simulink model "SPGF_FSK_0000_R2022b"  (R2022b)
settings: Solver=ode4  StartTime=0.0  StopTime=1.4  FixedStep=50e-6/50  RelTol=1e-3  EnableMultiTasking=on
undefined symbols (not defined in the file): D11, Delta
libraries: spsSeriesRLCBranchLib x1646, spsGroundLib x360, spsStairGeneratorLib x147, spsIdealSwitchLib x145, spsCurrentMeasurementLib x145, spsUniversalBridgeLib x76, spsThreePhaseSeriesRLCLoadLib x57, simulink x45, spsBistableLib x36, spsSequenceAnalyzerLib x31, spsThreePhaseParallelRLCLoadLib x20, spsThreePhaseTransformerTwoWindingsLib x20
(part 21 of 40)

== system SPGF_FSK_0000_R2022b/W15/concentrated ==
  Ccs/1 : spsSeriesRLCBranchLib/Series RLC Branch  LConnTagsString=__new0  RConnTagsString=__new0  BranchType=C  Resistance=190  Inductance=1e-3  SetiL0=off  InitialCurrent=0  Capacitance=-C_matrix(1,2)/2  Setx0=off  InitialVoltage=0  Measurements=None
  Ccs/2 : spsSeriesRLCBranchLib/Series RLC Branch  LConnTagsString=__new0  RConnTagsString=__new0  BranchType=C  Resistance=190  Inductance=1e-3  SetiL0=off  InitialCurrent=0  Capacitance=-C_matrix(1,2)/2  Setx0=off  InitialVoltage=0  Measurements=None
  Ccs2/1 : spsSeriesRLCBranchLib/Series RLC Branch  LConnTagsString=__new0  RConnTagsString=__new0  BranchType=C  Resistance=190  Inductance=1e-3  SetiL0=off  InitialCurrent=0  Capacitance=-C_matrix(3,4)/2  Setx0=off  InitialVoltage=0  Measurements=None
  Ccs2/2 : spsSeriesRLCBranchLib/Series RLC Branch  LConnTagsString=__new0  RConnTagsString=__new0  BranchType=C  Resistance=190  Inductance=1e-3  SetiL0=off  InitialCurrent=0  Capacitance=-C_matrix(3,4)/2  Setx0=off  InitialVoltage=0  Measurements=None
  Ccs2/3 : spsSeriesRLCBranchLib/Series RLC Branch  LConnTagsString=__new0  RConnTagsString=__new0  BranchType=R  Resistance=-Rg_matrix(3,4)*2  Inductance=1e-3  SetiL0=off  InitialCurrent=0  Capacitance=Rg_matrix(3,4)*2  Setx0=off  InitialVoltage=0  Measurements=None
  Ccs2/4 : spsSeriesRLCBranchLib/Series RLC Branch  LConnTagsString=__new0  RConnTagsString=__new0  BranchType=R  Resistance=-Rg_matrix(3,4)*2  Inductance=1e-3  SetiL0=off  InitialCurrent=0  Capacitance=Rg_matrix(3,4)*2  Setx0=off  InitialVoltage=0  Measurements=None
  Ccs3/1 : spsSeriesRLCBranchLib/Series RLC Branch  LConnTagsString=__new0  RConnTagsString=__new0  BranchType=C  Resistance=190  Inductance=1e-3  SetiL0=off  InitialCurrent=0  Capacitance=-C_matrix(5,6)/2  Setx0=off  InitialVoltage=0  Measurements=None
  Ccs3/2 : spsSeriesRLCBranchLib/Series RLC Branch  LConnTagsString=__new0  RConnTagsString=__new0  BranchType=C  Resistance=190  Inductance=1e-3  SetiL0=off  InitialCurrent=0  Capacitance=-C_matrix(5,6)/2  Setx0=off  InitialVoltage=0  Measurements=None
  Ccs3/3 : spsSeriesRLCBranchLib/Series RLC Branch  LConnTagsString=__new0  RConnTagsString=__new0  BranchType=R  Resistance=-Rg_matrix(5,6)*2  Inductance=1e-3  SetiL0=off  InitialCurrent=0  Capacitance=-C_matrix(5,6)/2  Setx0=off  InitialVoltage=0  Measurements=None
  Ccs3/4 : spsSeriesRLCBranchLib/Series RLC Branch  LConnTagsString=__new0  RConnTagsString=__new0  BranchType=R  Resistance=-Rg_matrix(5,6)*2  Inductance=1e-3  SetiL0=off  InitialCurrent=0  Capacitance=-C_matrix(5,6)/2  Setx0=off  InitialVoltage=0  Measurements=None
  Csg/2 : spsSeriesRLCBranchLib/Series RLC Branch  LConnTagsString=__new0  RConnTagsString=__new0  BranchType=C  Resistance=190  Inductance=1e-3  SetiL0=off  InitialCurrent=0  Capacitance=( C_matrix(1,2) + C_matrix(2,2) )/2  Setx0=off  InitialVoltage=0  Measurements=None
  Csg1/1 : spsSeriesRLCBranchLib/Series RLC Branch  LConnTagsString=__new0  RConnTagsString=__new0  BranchType=C  Resistance=190  Inductance=1e-3  SetiL0=off  InitialCurrent=0  Capacitance=( C_matrix(1,2) + C_matrix(2,2) )/2  Setx0=off  InitialVoltage=0  Measurements=None
  Csg2/1 : spsSeriesRLCBranchLib/Series RLC Branch  LConnTagsString=__new0  RConnTagsString=__new0  BranchType=C  Resistance=190  Inductance=1e-3  SetiL0=off  InitialCurrent=0  Capacitance=( C_matrix(3,4) + C_matrix(4,4) )/2  Setx0=off  InitialVoltage=0  Measurements=None
  Csg2/2 : spsSeriesRLCBranchLib/Series RLC Branch  LConnTagsString=__new0  RConnTagsString=__new0  BranchType=C  Resistance=190  Inductance=1e-3  SetiL0=off  InitialCurrent=0  Capacitance=( C_matrix(3,4) + C_matrix(4,4) )/2  Setx0=off  InitialVoltage=0  Measurements=None
  Csg3/1 : spsSeriesRLCBranchLib/Series RLC Branch  LConnTagsString=__new0  RConnTagsString=__new0  BranchType=C  Resistance=190  Inductance=1e-3  SetiL0=off  InitialCurrent=0  Capacitance=( C_matrix(5,6) + C_matrix(6,6) ) /2  Setx0=off  InitialVoltage=0  Measurements=None
  Csg3/2 : spsSeriesRLCBranchLib/Series RLC Branch  LConnTagsString=__new0  RConnTagsString=__new0  BranchType=C  Resistance=190  Inductance=1e-3  SetiL0=off  InitialCurrent=0  Capacitance=( C_matrix(5,6) + C_matrix(6,6) ) /2  Setx0=off  InitialVoltage=0  Measurements=None
  Ground{1..4} (4 alike) : spsGroundLib/Ground  LConnTagsString=a
  RL : spsMutualInductanceLib/Mutual Inductance  LConnTagsString=a|b|c|L4|L5|L6  RConnTagsString=A|B|C|R4|R5|R6  TypeOfMutual=Generalized mutual inductance  NumberOfWindings=6  SelfImpedance1=[1.1 1.1e-03]  SelfImpedance2=[ 1.1 1.1e-03]  ThreeWindings=on  SelfImpedance3=[ 1.1 1.1e-03]  MutualImpedance=[1.0 1.0e-03]  InductanceMatrix=L_matrix  ResistanceMatrix=R_matrix  Measurements=None
      settings: LibrarySourceBlock=sps_lib/Passives/Mutual Inductance
  Rcs*2 : spsSeriesRLCBranchLib/Series RLC Branch  LConnTagsString=__new0  RConnTagsString=__new0  BranchType=R  Resistance=-Rg_matrix(1,2)*2  Inductance=1e-3  SetiL0=off  InitialCurrent=0  Capacitance=Rg_matrix(1,2)*2  Setx0=off  InitialVoltage=0  Measurements=None
  Rgcs1/1 : spsSeriesRLCBranchLib/Series RLC Branch  LConnTagsString=__new0  RConnTagsString=__new0  BranchType=R  Resistance=-Rg_matrix(1,2)*2  Inductance=1e-3  SetiL0=off  InitialCurrent=0  Capacitance=Rg_matrix(1,2)*2  Setx0=off  InitialVoltage=0  Measurements=None
  Rgsg1/1 : spsSeriesRLCBranchLib/Series RLC Branch  LConnTagsString=__new0  RConnTagsString=__new0  BranchType=R  Resistance=(Rg_matrix(4,4)+Rg_matrix(3,4))*2  Inductance=1e-3  SetiL0=off  InitialCurrent=0  Capacitance=Rg_matrix(1,2)*2  Setx0=off  InitialVoltage=0  Measurements=None
  Rgsg1/2 : spsSeriesRLCBranchLib/Series RLC Branch  LConnTagsString=__new0  RConnTagsString=__new0  BranchType=R  Resistance=(Rg_matrix(2,2)+Rg_matrix(1,2))*2  Inductance=1e-3  SetiL0=off  InitialCurrent=0  Capacitance=Rg_matrix(1,2)*2  Setx0=off  InitialVoltage=0  Measurements=None
  Rgsg1/3 : spsSeriesRLCBranchLib/Series RLC Branch  LConnTagsString=__new0  RConnTagsString=__new0  BranchType=R  Resistance=(Rg_matrix(4,4)+Rg_matrix(3,4))*2  Inductance=1e-3  SetiL0=off  InitialCurrent=0  Capacitance=Rg_matrix(1,2)*2  Setx0=off  InitialVoltage=0  Measurements=None
  Rgsg1/4 : spsSeriesRLCBranchLib/Series RLC Branch  LConnTagsString=__new0  RConnTagsString=__new0  BranchType=R  Resistance=(Rg_matrix(2,2)+Rg_matrix(1,2))*2  Inductance=1e-3  SetiL0=off  InitialCurrent=0  Capacitance=Rg_matrix(1,2)*2  Setx0=off  InitialVoltage=0  Measurements=None
  Rsg*2 : spsSeriesRLCBranchLib/Series RLC Branch  LConnTagsString=__new0  RConnTagsString=__new0  BranchType=R  Resistance=(Rg_matrix(6,6)+Rg_matrix(5,6))*2  Inductance=1e-3  SetiL0=off  InitialCurrent=0  Capacitance=Rg_matrix(1,2)*2  Setx0=off  InitialVoltage=0  Measurements=None
  Rsg1/1 : spsSeriesRLCBranchLib/Series RLC Branch  LConnTagsString=__new0  RConnTagsString=__new0  BranchType=R  Resistance=(Rg_matrix(6,6)+Rg_matrix(5,6))*2  Inductance=1e-3  SetiL0=off  InitialCurrent=0  Capacitance=Rg_matrix(1,2)*2  Setx0=off  InitialVoltage=0  Measurements=None
  A : PMIOPort  Side=Left
  B : PMIOPort  Port=2  Side=Left
  C : PMIOPort  Port=3  Side=Left
  a : PMIOPort  Port=4  Side=Right
  b : PMIOPort  Port=5  Side=Right
  c : PMIOPort  Port=6  Side=Right
  connections:
  Ccs3/3/RConn1 -- RL/LConn5 -- C/RConn1 -- Ccs3/2/RConn1
  Ccs2/2/RConn1 -- Ccs2/3/RConn1 -- B/RConn1 -- RL/LConn3
  Ccs/2/RConn1 -- Rcs*2/RConn1 -- A/RConn1 -- RL/LConn1
  Ccs3/4/RConn1 -- RL/RConn5 -- c/RConn1 -- Ccs3/1/RConn1
  Ccs2/1/RConn1 -- Ccs2/4/RConn1 -- RL/RConn3 -- b/RConn1
  Ccs/1/RConn1 -- Rgcs1/1/RConn1 -- RL/RConn1 -- a/RConn1
  Csg/2/RConn1 -- Ground1/LConn1 -- Csg2/2/RConn1 -- Csg3/2/RConn1 -- Rgsg1/2/RConn1 -- Rgsg1/1/RConn1 -- Rsg*2/RConn1
  Csg3/1/LConn1 -- Ccs3/4/LConn1 -- Rsg1/1/LConn1 -- Ccs3/1/LConn1 -- RL/RConn6 -- Ground4/LConn1 -- RL/RConn2 -- Ccs/1/LConn1 -- Csg1/1/LConn1 -- Rgcs1/1/LConn1 -- Rgsg1/4/LConn1 -- RL/RConn4 -- Ccs2/1/LConn1 -- Csg2/1/LConn1 -- Ccs2/4/LConn1 -- Rgsg1/3/LConn1
  Csg1/1/RConn1 -- Ground2/LConn1 -- Csg2/1/RConn1 -- Csg3/1/RConn1 -- Rgsg1/4/RConn1 -- Rgsg1/3/RConn1 -- Rsg1/1/RConn1
  Ccs3/2/LConn1 -- Ccs3/3/LConn1 -- Csg3/2/LConn1 -- Rsg*2/LConn1 -- Ccs2/2/LConn1 -- Ccs2/3/LConn1 -- Csg2/2/LConn1 -- Rgsg1/1/LConn1 -- RL/LConn4 -- RL/LConn2 -- Ccs/2/LConn1 -- Rcs*2/LConn1 -- Csg/2/LConn1 -- Rgsg1/2/LConn1 -- Ground3/LConn1 -- RL/LConn6

== system SPGF_FSK_0000_R2022b/W21/DPL ==
  Ccs2/1 : spsSeriesRLCBranchLib/Series RLC Branch  LConnTagsString=__new0  RConnTagsString=__new0  BranchType=R  Resistance=-Rg_matrix(3,4)*2  Inductance=1e-3  SetiL0=off  InitialCurrent=0  Capacitance=Rg_matrix(3,4)*2  Setx0=off  InitialVoltage=0  Measurements=None
  Ccs2/3 : spsSeriesRLCBranchLib/Series RLC Branch  LConnTagsString=__new0  RConnTagsString=__new0  BranchType=R  Resistance=-Rg_matrix(3,4)*2  Inductance=1e-3  SetiL0=off  InitialCurrent=0  Capacitance=Rg_matrix(3,4)*2  Setx0=off  InitialVoltage=0  Measurements=None
  Ccs3/1 : spsSeriesRLCBranchLib/Series RLC Branch  LConnTagsString=__new0  RConnTagsString=__new0  BranchType=R  Resistance=-Rg_matrix(5,6)*2  Inductance=1e-3  SetiL0=off  InitialCurrent=0  Capacitance=-C_matrix(5,6)/2  Setx0=off  InitialVoltage=0  Measurements=None
  Ccs3/3 : spsSeriesRLCBranchLib/Series RLC Branch  LConnTagsString=__new0  RConnTagsString=__new0  BranchType=R  Resistance=-Rg_matrix(5,6)*2  Inductance=1e-3  SetiL0=off  InitialCurrent=0  Capacitance=-C_matrix(5,6)/2  Setx0=off  InitialVoltage=0  Measurements=None
  DPL : spsDistributedParametersLineLib/Distributed Parameters Line  Phases=6  Length=LineLength  Frequency=Frequency  Resistance=R_matrix  Inductance=L_matrix  Capacitance=C_matrix  x1=[-2.8e-05 -1.16534888629937 5056.85583270413 0 -2770.28944118531 0 0;-2.75e-05 -1.16569158516128 5058.29147397259 0 -2771.07592630165 0 0;-2.7e-05 -1.1660342552609 5059.72699043271 0 -2771.86234304442 0 0;-2.65e-05 -1.16637689658978 5061.16238204907 0 -2772.64869139424 0 0;-2.6e-05 -1.16671950913946 5062.59764878626 0 -2773.43497133169 0 0;-2.55e-05 -1.16706209290149 5064.03279060886 0 -2774.22118283738 0 0;-2.5e-05 -1.16740464786742 5065.46780748145 0 -2775.00732589191 0 0;-2.45e-05 -1.16774717402879 5066.90269936864 0 -2775.79340047587 0 0;-2.4e-05 -1.16808967137715 5068.33746623502 0 -2776.57940656987 0 0;-2.35e-05 -1.16843213990406 5069.77210804518 0 -2777.36534415453 0 0;-2.3e-05 -1.16877457960107 5071.20662476372 0 -2778.15121321044 0 0;-2.25e-05 -1.16911699045971 5072.64101635526 0 -2778.93701371822 0 0;-2.2e-05 -1.16945937247155 5074.07528278441 0 -2779.72274565848 0 0;-2.15e-05 -1.16980172562814 5075.50942401576 0 -2780.50840901182 0 0;-2.1e-05 -1.17014404992102 5076.94344001393 0 -2781.29400375888 0 0;-2.05e-05 -1.17048634534176 5078.37733074355 0 -2782.07952988025 0 0;-2e-05 -1.1708286118819 5079.81109616923 0 -2782.86498735656 0 0;-1.95e-05 -1.17117084953301 5081.2447362556 0 -2783.65037616843 0 0;-1.9e-05 -1.17151305828664 5082.67825096728 0 -2784.43569629649 0 0;-1.85e-05 -1.17185523813434 5084.1116402689 0 -2785.22094772134 0 0;-1.8e-05 -1.17219738906767 5085.54490412509 0 -2786.00613042362 0 0;-1.75e-05 -1.17253951107819 5086.97804250049 0 -2786.79124438396 0 0;-1.7e-05 -1.17288160415745 5088.41105535974 0 -2787.57628958298 0 0;-1.65e-05 -1.17322366829702 5089.84394266748 0 -2788.36126600131 0 0;-1.6e-05 -1.17356570348846 5091.27670438835 0 -2789.14617361959 0 0;-1.55e-05 -1.17390770972333 5092.70934048701 0 -2789.93101241844 0 0;-1.5e-05 -1.17424968699318 5094.1418509281 0 -2790.7157823785 0 0;-1.45e-05 -1.17459163528959 5095.57423567628 0 -2791.50048348041 0 0;-1.4e-05 -1.1749335546041 5097.00649469621 0 -2792.28511570481 0 0;-1.35e-05 -1.1752754449283 5098.43862795254 0 -2793.06967903233 0 0;-1.3e-05 -1.17561730625373 5099.87063540994 0 -2793.85417344363 0 0;-1.25e-05 -1.17595913857198 5101.30251703308 0 -2794.63859891933 0 0;-1.2e-05 -1.17630094187459 5102.73427278662 0 -2795.42295544009 0 0;-1.15e-05 -1.17664271615314 5104.16590263524 0 -2796.20724298656 0 0;-1.1e-05 -1.17698446139919 5105.59740654362 0 -2796.99146153937 0 0;-1.05e-05 -1.17732617760432 5107.02878447643 0 -2797.77561107919 0 0;-1e-05 -1.17766786476009 5108.46003639835 0 -2798.55969158666 0 0;-9.5e-06 -1.17800952285806 5109.89116227408 0 -2799.34370304244 0 0;-9e-06 -1.17835115188982 5111.32216206829 0 -2800.12764542718 0 0;-8.5e-06 -1.17869275184693 5112.75303574569 0 -2800.91151872155 0 0;-8e-06 -1.17903432272096 5114.18378327096 0 -2801.69532290619 0 0;-7.5e-06 -1.17937586450349 5115.61440460881 0 -2802.47905796177 0 0;-7e-06 -1.17971737718608 5117.04489972393 0 -2803.26272386895 0 0;-6.5e-06 -1.18005886076032 5118.47526858103 0 -2804.04632060839 0 0;-6e-06 -1.18040031521776 5119.90551114481 0 -2804.82984816077 0 0;-5.5e-06 -1.18074174055 5121.33562737999 -12.6660829679671 -2805.61330650674 0 0;-5e-06 -1.1810831367486 5122.76561725128 -12.6698010202153 -2806.39669562698 0 0;-4.5e-06 -1.18142450380515 5124.19548072339 -12.6735187598487 -2807.18001550216 4987.30313046272 -9097.9489590017;-4e-06 -1.18176584171121 5125.62521776104 -12.6772361867756 -2807.96326611294 4986.86192214537 -9097.14409700584;-3.5e-06 -1.18210715045837 5127.05482832897 -12.6809533009042 -2808.74644744002 4986.42059078213 -9096.33901054695;-3e-06 -1.18244843003821 5128.48431239189 -12.6846701021429 -2809.52955946405 4985.9791363839 -9095.53369964489;-2.5e-06 -1.1827896804423 5129.91366991452 -12.6883865903998 -2810.31260216571 4985.53755896156 -9094.72816431953;-2e-06 -1.18313090166222 5131.34290086162 -12.6921027655834 -2811.09557552569 4985.09585852602 -9093.92240459075;-1.5e-06 -1.18347209368956 5132.7720051979 -12.6958186276018 -2811.87847952467 4984.65403508816 -9093.11642047843;-1e-06 -1.1838132565159 5134.20098288811 -12.6995341763636 -2812.66131414333 4984.2120886589 -9092.31021200245;-5e-07 -1.18415439013281 5135.62983389699 -12.7032494117768 -2813.44407936236 4983.77001924914 -9091.50377918271]  x2=[-2.8e-05 -1.16510912460452 5063.16244321356 0 -2773.74438176613 0 0;-2.75e-05 -1.16545352542046 5064.60090637248 0 -2774.53241279433 0 0;-2.7e-05 -1.16579789747999 5066.03924456738 0 -2775.32037536367 0 0;-2.65e-05 -1.1661422407746 5067.47745776277 0 -2776.10826945474 0 0;-2.6e-05 -1.16648655529581 5068.91554592317 0 -2776.89609504807 0 0;-2.55e-05 -1.16683084103512 5070.35350901309 0 -2777.68385212425 0 0;-2.5e-05 -1.16717509798403 5071.79134699705 0 -2778.47154066382 0 0;-2.45e-05 -1.16751932613405 5073.22905983957 0 -2779.25916064735 0 0;-2.4e-05 -1.16786352547669 5074.66664750519 0 -2780.04671205541 0 0;-2.35e-05 -1.16820769600344 5076.10410995842 0 -2780.83419486857 0 0;-2.3e-05 -1.16855183770583 5077.54144716381 0 -2781.6216090674 0 0;-2.25e-05 -1.16889595057536 5078.97865908588 0 -2782.40895463246 0 0;-2.2e-05 -1.16924003460353 5080.41574568918 0 -2783.19623154434 0 0;-2.15e-05 -1.16958408978187 5081.85270693825 0 -2783.9834397836 0 0;-2.1e-05 -1.16992811610187 5083.28954279763 0 -2784.77057933082 0 0;-2.05e-05 -1.17027211355506 5084.72625323186 0 -2785.55765016658 0 0;-2e-05 -1.17061608213293 5086.1628382055 0 -2786.34465227147 0 0;-1.95e-05 -1.17096002182702 5087.59929768311 0 -2787.13158562605 0 0;-1.9e-05 -1.17130393262882 5089.03563162923 0 -2787.91845021092 0 0;-1.85e-05 -1.17164781452986 5090.47184000843 0 -2788.70524600666 0 0;-1.8e-05 -1.17199166752164 5091.90792278528 0 -2789.49197299386 0 0;-1.75e-05 -1.17233549159569 5093.34387992433 0 -2790.2786311531 0 0;-1.7e-05 -1.17267928674353 5094.77971139016 0 -2791.06522046497 0 0;-1.65e-05 -1.17302305295666 5096.21541714735 0 -2791.85174091007 0 0;-1.6e-05 -1.1733667902266 5097.65099716045 0 -2792.63819246899 0 0;-1.55e-05 -1.17371049854489 5099.08645139406 0 -2793.42457512233 0 0;-1.5e-05 -1.17405417790302 5100.52177981275 0 -2794.21088885067 0 0;-1.45e-05 -1.17439782829253 5101.95698238112 0 -2794.99713363463 0 0;-1.4e-05 -1.17474144970494 5103.39205906374 0 -2795.78330945479 0 0;-1.35e-05 -1.17508504213176 5104.82700982521 0 -2796.56941629177 0 0;-1.3e-05 -1.17542860556452 5106.26183463012 0 -2797.35545412617 0 0;-1.25e-05 -1.17577213999474 5107.69653344307 0 -2798.14142293858 0 0;-1.2e-05 -1.17611564541395 5109.13110622866 0 -2798.92732270962 0 0;-1.15e-05 -1.17645912181367 5110.5655529515 0 -2799.7131534199 0 0;-1.1e-05 -1.17680256918542 5111.99987357618 0 -2800.49891505003 0 0;-1.05e-05 -1.17714598752073 5113.43406806733 0 -2801.28460758061 0 0;-1e-05 -1.17748937681113 5114.86813638954 0 -2802.07023099227 0 0;-9.5e-06 -1.17783273704815 5116.30207850745 0 -2802.85578526562 0 0;-9e-06 -1.1781760682233 5117.73589438565 0 -2803.64127038127 0 0;-8.5e-06 -1.17851937032813 5119.16958398879 0 -2804.42668631985 0 0;-8e-06 -1.17886264335416 5120.60314728148 0 -2805.21203306197 0 0;-7.5e-06 -1.17920588729292 5122.03658422836 0 -2805.99731058826 0 0;-7e-06 -1.17954910213593 5123.46989479404 0 -2806.78251887934 0 0;-6.5e-06 -1.17989228787475 5124.90307894318 0 -2807.56765791584 0 0;-6e-06 -1.18023544450088 5126.3361366404 0 -2808.35272767838 0 0;-5.5e-06 -1.18057857200588 5127.76906785034 -12.6564826349605 -2809.1377281476 0 0;-5e-06 -1.18092167038126 5129.20187253766 -12.6602239684602 -2809.92265930412 0 0;-4.5e-06 -1.18126473961857 5130.63455066699 -12.6639649895814 -2810.70752112858 4996.71752818238 -9115.12291207668;-4e-06 -1.18160777970934 5132.06710220299 -12.6677056982318 -2811.49231360161 4996.27596698537 -9114.31740634991;-3.5e-06 -1.18195079064511 5133.49952711031 -12.6714460943191 -2812.27703670385 4995.83428251018 -9113.51167573637;-3e-06 -1.18229377241741 5134.9318253536 -12.675186177751 -2813.06169041594 4995.39247476773 -9112.70572025595;-2.5e-06 -1.18263672501778 5136.36399689754 -12.6789259484352 -2813.84627471851 4994.95054376891 -9111.89953992853;-2e-06 -1.18297964843776 5137.79604170677 -12.6826654062795 -2814.6307895922 4994.50848952462 -9111.09313477399;-1.5e-06 -1.18332254266889 5139.22795974596 -12.6864045511915 -2815.41523501767 4994.06631204578 -9110.28650481225;-1e-06 -1.18366540770271 5140.65975097979 -12.6901433830791 -2816.19961097555 4993.62401134329 -9109.4796500632;-5e-07 -1.18400824353075 5142.09141537292 -12.6938819018499 -2816.98391744649 4993.18158742807 -9108.67257054674]  x3=[-2.8e-05 -4.26783627359743e-06 43.4620546748687 0 -260.320398510763 0 0;-2.75e-05 -6.64716416284354e-06 43.4958297492458 0 -260.396991199751 0 0;-2.7e-05 -9.0264918880775e-06 43.5296037504063 0 -260.473577463702 0 0;-2.65e-05 -1.14058193905917e-05 43.5633766775169 0 -260.550157300724 0 0;-2.6e-05 -1.37851466116785e-05 43.5971485297442 0 -260.626730708929 0 0;-2.55e-05 -1.61644734926305e-05 43.630919306255 0 -260.703297686428 0 0;-2.5e-05 -1.85437999747402e-05 43.664689006216 0 -260.77985823133 0 0;-2.45e-05 -2.09231259992999e-05 43.6984576287941 0 -260.856412341747 0 0;-2.4e-05 -2.33024515076021e-05 43.7322251731559 0 -260.93296001579 0 0;-2.35e-05 -2.56817764409394e-05 43.7659916384683 0 -261.00950125157 0 0;-2.3e-05 -2.80611007406043e-05 43.7997570238981 0 -261.0860360472 0 0;-2.25e-05 -3.04404243478893e-05 43.8335213286123 0 -261.162564400789 0 0;-2.2e-05 -3.28197472040869e-05 43.8672845517776 0 -261.23908631045 0 0;-2.15e-05 -3.51990692504896e-05 43.9010466925612 0 -261.315601774296 0 0;-2.1e-05 -3.75783904283902e-05 43.9348077501298 0 -261.392110790437 0 0;-2.05e-05 -3.99577106790812e-05 43.9685677236505 0 -261.468613356987 0 0;-2e-05 -4.23370299438552e-05 44.0023266122902 0 -261.545109472057 0 0;-1.95e-05 -4.47163481640048e-05 44.0360844152161 0 -261.62159913376 0 0;-1.9e-05 -4.70956652808228e-05 44.0698411315951 0 -261.698082340209 0 0;-1.85e-05 -4.94749812356017e-05 44.1035967605944 0 -261.774559089517 0 0;-1.8e-05 -5.18542959696346e-05 44.1373513013811 0 -261.851029379796 0 0;-1.75e-05 -5.42336094242139e-05 44.1711047531223 0 -261.92749320916 0 0;-1.7e-05 -5.66129215406325e-05 44.2048571149851 0 -262.003950575723 0 0;-1.65e-05 -5.89922322601833e-05 44.2386083861368 0 -262.080401477597 0 0;-1.6e-05 -6.13715415241591e-05 44.2723585657447 0 -262.156845912896 0 0;-1.55e-05 -6.37508492738528e-05 44.3061076529758 0 -262.233283879734 0 0;-1.5e-05 -6.61301554505574e-05 44.3398556469976 0 -262.309715376226 0 0;-1.45e-05 -6.85094599955658e-05 44.3736025469773 0 -262.386140400484 0 0;-1.4e-05 -7.0888762850171e-05 44.4073483520822 0 -262.462558950625 0 0;-1.35e-05 -7.32680639556661e-05 44.4410930614798 0 -262.538971024761 0 0;-1.3e-05 -7.56473632533442e-05 44.4748366743373 0 -262.615376621007 0 0;-1.25e-05 -7.80266606844984e-05 44.5085791898222 0 -262.691775737479 0 0;-1.2e-05 -8.0405956190422e-05 44.5423206071019 0 -262.768168372292 0 0;-1.15e-05 -8.27852497124081e-05 44.576060925344 0 -262.844554523559 0 0;-1.1e-05 -8.516454119175e-05 44.6098001437158 0 -262.920934189397 0 0;-1.05e-05 -8.75438305697411e-05 44.6435382613849 0 -262.997307367922 0 0;-1e-05 -8.99231177876749e-05 44.6772752775189 0 -263.073674057247 0 0;-9.5e-06 -9.23024027868445e-05 44.7110111912853 0 -263.15003425549 0 0;-9e-06 -9.46816855085437e-05 44.7447460018517 0 -263.226387960766 0 0;-8.5e-06 -9.7060965894066e-05 44.7784797083857 0 -263.302735171192 0 0;-8e-06 -9.94402438847049e-05 44.8122123100551 0 -263.379075884883 0 0;-7.5e-06 -0.000101819519421754 44.8459438060274 0 -263.455410099955 0 0;-7e-06 -0.000104198792446507 44.8796741954705 0 -263.531737814526 0 0;-6.5e-06 -0.000106578062900259 44.9134034775519 0 -263.608059026712 0 0;-6e-06 -0.000108957330724302 44.9471316514396 0 -263.68437373463 0 0;-5.5e-06 -0.00011133659585993 44.9808587163012 -0.835958382231405 -263.760681936397 0 0;-5e-06 -0.000113715858248438 45.0145846713046 -0.836322757975905 -263.83698363013 0 0;-4.5e-06 -0.00011609511783112 45.0483095156177 -0.836687113084968 -263.913278813946 514.841663054707 -236.599753323224;-4e-06 -0.00011847437454927 45.0820332484083 -0.837051447549604 -263.989567485963 514.798101260749 -236.590465344622;-3.5e-06 -0.000120853628344181 45.1157558688443 -0.837415761360824 -264.065849644298 514.754526764657 -236.581171528384;-3e-06 -0.000123232879157149 45.1494773760937 -0.837780054509638 -264.14212528707 514.710939567506 -236.571871874739;-2.5e-06 -0.000125612126929467 45.1831977693243 -0.838144326987057 -264.218394412396 514.667339670372 -236.562566383918 ...(+471 chars)]  x4=[-2.8e-05 -0.0140226628107478 91.5383252097823 0 -240.863301074738 0 0;-2.75e-05 -0.0140244628801063 91.5429574729256 0 -240.929298928784 0 0;-2.7e-05 -0.0140262626034252 91.5475874773368 0 -240.995290838137 0 0;-2.65e-05 -0.0140280619806598 91.552215222902 0 -241.061276801169 0 0;-2.6e-05 -0.0140298610117659 91.5568407095068 0 -241.127256816253 0 0;-2.55e-05 -0.0140316596966991 91.561463937037 0 -241.193230881761 0 0;-2.5e-05 -0.014033458035415 91.5660849053787 0 -241.259198996064 0 0;-2.45e-05 -0.0140352560278691 91.5707036144179 0 -241.325161157535 0 0;-2.4e-05 -0.0140370536740172 91.5753200640405 0 -241.391117364546 0 0;-2.35e-05 -0.0140388509738149 91.5799342541326 0 -241.45706761547 0 0;-2.3e-05 -0.0140406479272178 91.5845461845804 0 -241.52301190868 0 0;-2.25e-05 -0.0140424445341816 91.5891558552702 0 -241.588950242549 0 0;-2.2e-05 -0.014044240794662 91.5937632660881 0 -241.654882615449 0 0;-2.15e-05 -0.0140460367086146 91.5983684169205 0 -241.720809025754 0 0;-2.1e-05 -0.0140478322759951 91.6029713076537 0 -241.786729471837 0 0;-2.05e-05 -0.0140496274967593 91.6075719381743 0 -241.852643952071 0 0;-2e-05 -0.0140514223708629 91.6121703083685 0 -241.918552464831 0 0;-1.95e-05 -0.0140532168982615 91.6167664181231 0 -241.984455008489 0 0;-1.9e-05 -0.0140550110789108 91.6213602673247 0 -242.050351581421 0 0;-1.85e-05 -0.0140568049127667 91.6259518558597 0 -242.116242182 0 0;-1.8e-05 -0.0140585983997848 91.630541183615 0 -242.182126808599 0 0;-1.75e-05 -0.0140603915399209 91.6351282504774 0 -242.248005459595 0 0;-1.7e-05 -0.0140621843331307 91.6397130563335 0 -242.31387813336 0 0;-1.65e-05 -0.01406397677937 91.6442956010704 0 -242.37974482827 0 0;-1.6e-05 -0.0140657688785947 91.648875884575 0 -242.4456055427 0 0;-1.55e-05 -0.0140675606307603 91.6534539067342 0 -242.511460275024 0 0;-1.5e-05 -0.0140693520358229 91.658029667435 0 -242.577309023618 0 0;-1.45e-05 -0.0140711430937381 91.6626031665647 0 -242.643151786856 0 0;-1.4e-05 -0.0140729338044618 91.6671744040102 0 -242.708988563115 0 0;-1.35e-05 -0.0140747241679497 91.6717433796589 0 -242.774819350769 0 0;-1.3e-05 -0.0140765141841577 91.676310093398 0 -242.840644148195 0 0;-1.25e-05 -0.0140783038530417 91.6808745451148 0 -242.906462953769 0 0;-1.2e-05 -0.0140800931745575 91.6854367346967 0 -242.972275765865 0 0;-1.15e-05 -0.0140818821486608 91.6899966620311 0 -243.038082582861 0 0;-1.1e-05 -0.0140836707753077 91.6945543270055 0 -243.103883403133 0 0;-1.05e-05 -0.0140854590544539 91.6991097295076 0 -243.169678225056 0 0;-1e-05 -0.0140872469860554 91.7036628694247 0 -243.235467047009 0 0;-9.5e-06 -0.0140890345700679 91.7082137466447 0 -243.301249867366 0 0;-9e-06 -0.0140908218064475 91.7127623610553 0 -243.367026684507 0 0;-8.5e-06 -0.01409260869515 91.7173087125441 0 -243.432797496806 0 0;-8e-06 -0.0140943952361313 91.721852800999 0 -243.498562302642 0 0;-7.5e-06 -0.0140961814293473 91.726394626308 0 -243.564321100392 0 0;-7e-06 -0.014097967274754 91.7309341883588 0 -243.630073888433 0 0;-6.5e-06 -0.0140997527723073 91.7354714870396 0 -243.695820665142 0 0;-6e-06 -0.0141015379219631 91.7400065222384 0 -243.761561428899 0 0;-5.5e-06 -0.0141033227236775 91.7445392938432 -1.0186771696074 -243.82729617808 0 0;-5e-06 -0.0141051071774063 91.7490698017423 -1.01886024502449 -243.893024911064 0 0;-4.5e-06 -0.0141068912831055 91.7535980458238 -1.01904329530221 -243.958747626228 450.89936877339 -48.814783490625;-4e-06 -0.0141086750407311 91.7581240259761 -1.01922632043605 -244.024464321952 450.857682085038 -48.7988728473647;-3.5e-06 -0.0141104584502392 91.7626477420874 -1.01940932042148 -244.090174996614 450.815984272219 -48.7829610000405;-3e-06 -0.0141122415115856 91.7671691940461 -1.019592295254 -244.155879648591 450.774275335962 -48.767047949045;-2.5e-06 -0.0141140242247264 91.7716883817406 -1.01977524492909 -244.221578276264 450.732555277295 -48.7511336947708;-2e-06 -0.0141158065896177 91.7762053050596 -1.01995816944223 -244.287270878011 450.690824097248 -48.7352182376106;-1.5e-06 -0.0141175886062154 91.7807199638914 -1.02014106878891 -244.352957452212 450.649081796851 -48.7193015779571;-1e-06 -0.0141193702744755 91.7852323581247 -1.02032394296462 -244.418637997244 450.607328377133 -48.7033837162031;-5e-07 -0.0141211515943542 91.7897424876483 -1.02050679196485 -244.484312511489 450.565563839125 -48.6874646527412]  x5=2.77139177619252e-05  V1=ones(3,3)  V2=ones(3,3)  I1=ones(3,3)  I2=ones(3,3)  nHarmo=1  Measurements=None  Decoupling=off  VsMag0=0  VrMag0=0  VsAngle0=0  VrAngle0=0  IsMag0=0  IrMag0=0  IsAngle0=0  IrAngle0=0
      settings: LibrarySourceBlock=sps_lib/Power Grid Elements/Distributed Parameters Line
  Ground{1..4} (4 alike) : spsGroundLib/Ground  LConnTagsString=a
  Rcs*1 : spsSeriesRLCBranchLib/Series RLC Branch  LConnTagsString=__new0  RConnTagsString=__new0  BranchType=R  Resistance=-Rg_matrix(1,2)*2  Inductance=1e-3  SetiL0=off  InitialCurrent=0  Capacitance=Rg_matrix(1,2)*2  Setx0=off  InitialVoltage=0  Measurements=None
  Rcs*2 : spsSeriesRLCBranchLib/Series RLC Branch  LConnTagsString=__new0  RConnTagsString=__new0  BranchType=R  Resistance=-Rg_matrix(1,2)*2  Inductance=1e-3  SetiL0=off  InitialCurrent=0  Capacitance=Rg_matrix(1,2)*2  Setx0=off  InitialVoltage=0  Measurements=None
  Rgsg1/1 : spsSeriesRLCBranchLib/Series RLC Branch  LConnTagsString=__new0  RConnTagsString=__new0  BranchType=R  Resistance=(Rg_matrix(4,4)+Rg_matrix(3,4))*2  Inductance=1e-3  SetiL0=off  InitialCurrent=0  Capacitance=Rg_matrix(1,2)*2  Setx0=off  InitialVoltage=0  Measurements=None
  Rgsg1/2 : spsSeriesRLCBranchLib/Series RLC Branch  LConnTagsString=__new0  RConnTagsString=__new0  BranchType=R  Resistance=(Rg_matrix(2,2)+Rg_matrix(1,2))*2  Inductance=1e-3  SetiL0=off  InitialCurrent=0  Capacitance=Rg_matrix(1,2)*2  Setx0=off  InitialVoltage=0  Measurements=None
  Rgsg1/3 : spsSeriesRLCBranchLib/Series RLC Branch  LConnTagsString=__new0  RConnTagsString=__new0  BranchType=R  Resistance=(Rg_matrix(4,4)+Rg_matrix(3,4))*2  Inductance=1e-3  SetiL0=off  InitialCurrent=0  Capacitance=Rg_matrix(1,2)*2  Setx0=off  InitialVoltage=0  Measurements=None
  Rgsg1/4 : spsSeriesRLCBranchLib/Series RLC Branch  LConnTagsString=__new0  RConnTagsString=__new0  BranchType=R  Resistance=(Rg_matrix(2,2)+Rg_matrix(1,2))*2  Inductance=1e-3  SetiL0=off  InitialCurrent=0  Capacitance=Rg_matrix(1,2)*2  Setx0=off  InitialVoltage=0  Measurements=None
  Rsg*1 : spsSeriesRLCBranchLib/Series RLC Branch  LConnTagsString=__new0  RConnTagsString=__new0  BranchType=R  Resistance=(Rg_matrix(6,6)+Rg_matrix(5,6))*2  Inductance=1e-3  SetiL0=off  InitialCurrent=0  Capacitance=Rg_matrix(1,2)*2  Setx0=off  InitialVoltage=0  Measurements=None
  Rsg*2 : spsSeriesRLCBranchLib/Series RLC Branch  LConnTagsString=__new0  RConnTagsString=__new0  BranchType=R  Resistance=(Rg_matrix(6,6)+Rg_matrix(5,6))*2  Inductance=1e-3  SetiL0=off  InitialCurrent=0  Capacitance=Rg_matrix(1,2)*2  Setx0=off  InitialVoltage=0  Measurements=None
  A : PMIOPort  Side=Left
  B : PMIOPort  Port=2  Side=Left
  C : PMIOPort  Port=3  Side=Left
  a : PMIOPort  Port=4  Side=Right
  b : PMIOPort  Port=5  Side=Right
  c : PMIOPort  Port=6  Side=Right
  connections:
  A/RConn1 -- DPL/LConn1 -- Rcs*2/RConn1
  B/RConn1 -- DPL/LConn3 -- Ccs2/3/RConn1
  C/RConn1 -- DPL/LConn5 -- Ccs3/3/RConn1
  Rgsg1/2/RConn1 -- Rsg*2/RConn1 -- Rgsg1/1/RConn1 -- Ground2/LConn1
  DPL/LConn2 -- Rcs*2/LConn1 -- Rgsg1/2/LConn1 -- DPL/LConn4 -- Ccs2/3/LConn1 -- Rgsg1/1/LConn1 -- DPL/LConn6 -- Rsg*2/LConn1 -- Ccs3/3/LConn1 -- Ground3/LConn1
  Rgsg1/3/RConn1 -- Rsg*1/RConn1 -- Rgsg1/4/RConn1 -- Ground1/LConn1
  Rgsg1/3/LConn1 -- Ccs2/1/LConn1 -- DPL/RConn4 -- DPL/RConn2 -- Rgsg1/4/LConn1 -- Rcs*1/LConn1 -- Rsg*1/LConn1 -- Ccs3/1/LConn1 -- DPL/RConn6 -- Ground4/LConn1
  Rcs*1/RConn1 -- DPL/RConn1 -- a/RConn1
  DPL/RConn3 -- Ccs2/1/RConn1 -- b/RConn1
  DPL/RConn5 -- Ccs3/1/RConn1 -- c/RConn1

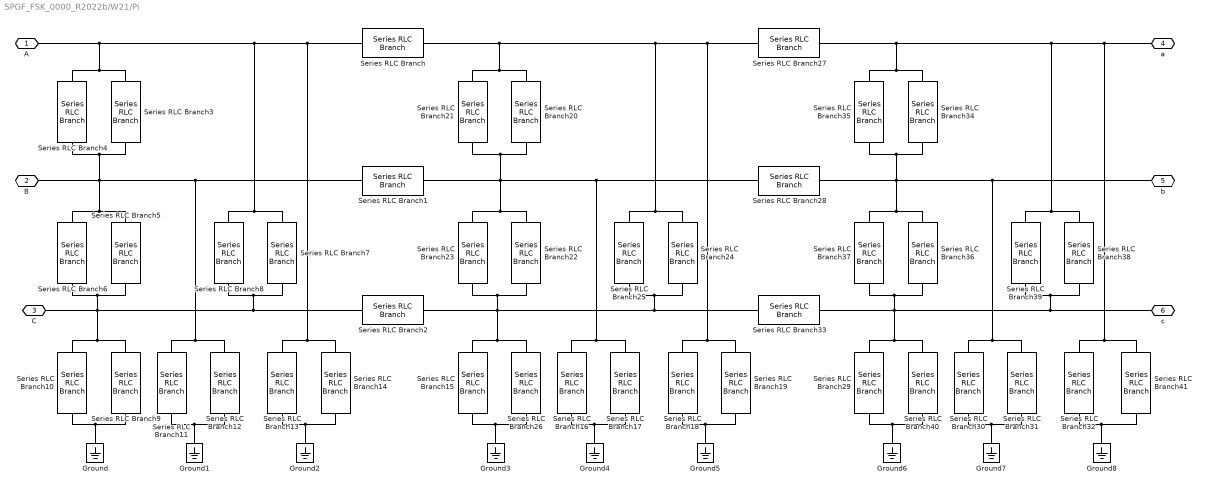
== system SPGF_FSK_0000_R2022b/W21/Pi ==
  Ground{,1..8} (9 alike) : spsGroundLib/Ground  LConnTagsString=a
  Series RLC Branch{,1..2,27..28,33} (6 alike) : spsSeriesRLCBranchLib/Series RLC Branch  LConnTagsString=__new0  RConnTagsString=__new0  BranchType=RL  Resistance=R/2  Inductance=L/2  SetiL0=off  InitialCurrent=0  Capacitance=1e-6  Setx0=off  InitialVoltage=0  Measurements=None
  Series RLC Branch{10..11,13,29..30,32} (6 alike) : spsSeriesRLCBranchLib/Series RLC Branch  LConnTagsString=__new0  RConnTagsString=__new0  BranchType=R  Resistance=Rfg*4  Inductance=L/2  SetiL0=off  InitialCurrent=0  Capacitance=1e-6  Setx0=off  InitialVoltage=0  Measurements=None
  Series RLC Branch{9,12,14,31,40..41} (6 alike) : spsSeriesRLCBranchLib/Series RLC Branch  LConnTagsString=__new0  RConnTagsString=__new0  BranchType=C  Resistance=R/2  Inductance=L/2  SetiL0=off  InitialCurrent=0  Capacitance=Cfg*0.25  Setx0=off  InitialVoltage=0  Measurements=None
  Series RLC Branch15 : spsSeriesRLCBranchLib/Series RLC Branch  LConnTagsString=__new0  RConnTagsString=__new0  BranchType=R  Resistance=Rfg*2  Inductance=L/2  SetiL0=off  InitialCurrent=0  Capacitance=1e-6  Setx0=off  InitialVoltage=0  Measurements=None
  Series RLC Branch16 : spsSeriesRLCBranchLib/Series RLC Branch  LConnTagsString=__new0  RConnTagsString=__new0  BranchType=R  Resistance=Rfg*2  Inductance=L/2  SetiL0=off  InitialCurrent=0  Capacitance=1e-6  Setx0=off  InitialVoltage=0  Measurements=None
  Series RLC Branch17 : spsSeriesRLCBranchLib/Series RLC Branch  LConnTagsString=__new0  RConnTagsString=__new0  BranchType=C  Resistance=R/2  Inductance=L/2  SetiL0=off  InitialCurrent=0  Capacitance=Cfg*0.5  Setx0=off  InitialVoltage=0  Measurements=None
  Series RLC Branch18 : spsSeriesRLCBranchLib/Series RLC Branch  LConnTagsString=__new0  RConnTagsString=__new0  BranchType=R  Resistance=Rfg*2  Inductance=L/2  SetiL0=off  InitialCurrent=0  Capacitance=1e-6  Setx0=off  InitialVoltage=0  Measurements=None
  Series RLC Branch19 : spsSeriesRLCBranchLib/Series RLC Branch  LConnTagsString=__new0  RConnTagsString=__new0  BranchType=C  Resistance=R/2  Inductance=L/2  SetiL0=off  InitialCurrent=0  Capacitance=Cfg*0.5  Setx0=off  InitialVoltage=0  Measurements=None
  Series RLC Branch20 : spsSeriesRLCBranchLib/Series RLC Branch  LConnTagsString=__new0  RConnTagsString=__new0  BranchType=C  Resistance=R/2  Inductance=L/2  SetiL0=off  InitialCurrent=0  Capacitance=Cmf*0.5  Setx0=off  InitialVoltage=0  Measurements=None
  Series RLC Branch21 : spsSeriesRLCBranchLib/Series RLC Branch  LConnTagsString=__new0  RConnTagsString=__new0  BranchType=R  Resistance=Rmf*2  Inductance=L/2  SetiL0=off  InitialCurrent=0  Capacitance=1e-6  Setx0=off  InitialVoltage=0  Measurements=None
  Series RLC Branch22 : spsSeriesRLCBranchLib/Series RLC Branch  LConnTagsString=__new0  RConnTagsString=__new0  BranchType=C  Resistance=R/2  Inductance=L/2  SetiL0=off  InitialCurrent=0  Capacitance=Cmf*0.5  Setx0=off  InitialVoltage=0  Measurements=None
  Series RLC Branch23 : spsSeriesRLCBranchLib/Series RLC Branch  LConnTagsString=__new0  RConnTagsString=__new0  BranchType=R  Resistance=Rmf*2  Inductance=L/2  SetiL0=off  InitialCurrent=0  Capacitance=1e-6  Setx0=off  InitialVoltage=0  Measurements=None
  Series RLC Branch24 : spsSeriesRLCBranchLib/Series RLC Branch  LConnTagsString=__new0  RConnTagsString=__new0  BranchType=C  Resistance=R/2  Inductance=L/2  SetiL0=off  InitialCurrent=0  Capacitance=Cmf*0.5  Setx0=off  InitialVoltage=0  Measurements=None
  Series RLC Branch25 : spsSeriesRLCBranchLib/Series RLC Branch  LConnTagsString=__new0  RConnTagsString=__new0  BranchType=R  Resistance=Rmf*2  Inductance=L/2  SetiL0=off  InitialCurrent=0  Capacitance=1e-6  Setx0=off  InitialVoltage=0  Measurements=None
  Series RLC Branch26 : spsSeriesRLCBranchLib/Series RLC Branch  LConnTagsString=__new0  RConnTagsString=__new0  BranchType=C  Resistance=R/2  Inductance=L/2  SetiL0=off  InitialCurrent=0  Capacitance=Cfg*0.5  Setx0=off  InitialVoltage=0  Measurements=None
  Series RLC Branch{3,5,7,34,36,38} (6 alike) : spsSeriesRLCBranchLib/Series RLC Branch  LConnTagsString=__new0  RConnTagsString=__new0  BranchType=C  Resistance=R/2  Inductance=L/2  SetiL0=off  InitialCurrent=0  Capacitance=Cmf*0.25  Setx0=off  InitialVoltage=0  Measurements=None
  Series RLC Branch{4,6,8,35,37,39} (6 alike) : spsSeriesRLCBranchLib/Series RLC Branch  LConnTagsString=__new0  RConnTagsString=__new0  BranchType=R  Resistance=Rmf*4  Inductance=L/2  SetiL0=off  InitialCurrent=0  Capacitance=1e-6  Setx0=off  InitialVoltage=0  Measurements=None
  A : PMIOPort  Side=Left
  B : PMIOPort  Port=2  Side=Left
  C : PMIOPort  Port=3  Side=Left
  a : PMIOPort  Port=4  Side=Right
  b : PMIOPort  Port=5  Side=Right
  c : PMIOPort  Port=6  Side=Right
  connections:
  Series RLC Branch12/LConn1 -- Series RLC Branch11/LConn1 -- Series RLC Branch5/LConn1 -- Series RLC Branch6/LConn1 -- B/RConn1 -- Series RLC Branch4/RConn1 -- Series RLC Branch3/RConn1 -- Series RLC Branch1/LConn1
  Series RLC Branch13/LConn1 -- A/RConn1 -- Series RLC Branch4/LConn1 -- Series RLC Branch3/LConn1 -- Series RLC Branch7/LConn1 -- Series RLC Branch8/LConn1 -- Series RLC Branch/LConn1 -- Series RLC Branch14/LConn1
  Series RLC Branch9/LConn1 -- Series RLC Branch2/LConn1 -- Series RLC Branch8/RConn1 -- Series RLC Branch7/RConn1 -- C/RConn1 -- Series RLC Branch5/RConn1 -- Series RLC Branch6/RConn1 -- Series RLC Branch10/LConn1
  Series RLC Branch9/RConn1 -- Ground/LConn1 -- Series RLC Branch10/RConn1
  Series RLC Branch12/RConn1 -- Series RLC Branch11/RConn1 -- Ground1/LConn1
  Series RLC Branch13/RConn1 -- Series RLC Branch14/RConn1 -- Ground2/LConn1
  Series RLC Branch17/LConn1 -- Series RLC Branch16/LConn1 -- Series RLC Branch28/LConn1 -- Series RLC Branch1/RConn1 -- Series RLC Branch23/LConn1 -- Series RLC Branch22/LConn1 -- Series RLC Branch20/RConn1 -- Series RLC Branch21/RConn1
  Series RLC Branch21/LConn1 -- Series RLC Branch20/LConn1 -- Series RLC Branch/RConn1 -- Series RLC Branch27/LConn1 -- Series RLC Branch19/LConn1 -- Series RLC Branch18/LConn1 -- Series RLC Branch24/LConn1 -- Series RLC Branch25/LConn1
  Series RLC Branch26/LConn1 -- Series RLC Branch15/LConn1 -- Series RLC Branch2/RConn1 -- Series RLC Branch33/LConn1 -- Series RLC Branch25/RConn1 -- Series RLC Branch24/RConn1 -- Series RLC Branch22/RConn1 -- Series RLC Branch23/RConn1
  Series RLC Branch26/RConn1 -- Series RLC Branch15/RConn1 -- Ground3/LConn1
  Ground4/LConn1 -- Series RLC Branch17/RConn1 -- Series RLC Branch16/RConn1
  Ground5/LConn1 -- Series RLC Branch18/RConn1 -- Series RLC Branch19/RConn1
  Series RLC Branch31/LConn1 -- b/RConn1 -- Series RLC Branch35/RConn1 -- Series RLC Branch34/RConn1 -- Series RLC Branch36/LConn1 -- Series RLC Branch37/LConn1 -- Series RLC Branch28/RConn1 -- Series RLC Branch30/LConn1
  Series RLC Branch34/LConn1 -- a/RConn1 -- Series RLC Branch41/LConn1 -- Series RLC Branch32/LConn1 -- Series RLC Branch38/LConn1 -- Series RLC Branch39/LConn1 -- Series RLC Branch27/RConn1 -- Series RLC Branch35/LConn1
  Series RLC Branch29/LConn1 -- Series RLC Branch36/RConn1 -- Series RLC Branch37/RConn1 -- c/RConn1 -- Series RLC Branch39/RConn1 -- Series RLC Branch38/RConn1 -- Series RLC Branch33/RConn1 -- Series RLC Branch40/LConn1
  Series RLC Branch29/RConn1 -- Series RLC Branch40/RConn1 -- Ground6/LConn1
  Series RLC Branch31/RConn1 -- Series RLC Branch30/RConn1 -- Ground7/LConn1
  Series RLC Branch32/RConn1 -- Series RLC Branch41/RConn1 -- Ground8/LConn1

== system SPGF_FSK_0000_R2022b/W21/Q ==
  breaker : Subsystem  Commented=on  mask{SwitchA=on, SwitchB=on, SwitchC=on, InitialStatus=[0 0 0], BreakerResistance=0.0001, SnubberResistance=1e6, SnubberCapacitance=inf, TransitionTimes=[0.2], ShiftTimes=[0 0.02 0.04]}
      mask prompts: SwitchA "Switching of phase A"; SwitchB "Switching of phase B"; SwitchC "Switching of phase C"; InitialStatus "Initial status of phase breaker [A, B, C]"; BreakerResistance "Breaker resistance Ron (ohms) :"; SnubberResistance "Snubbers resistance Rp (ohms) :"; SnubberCapacitance "Snubbers capacitance Cp (F) :"; TransitionTimes "Transition times (s) :"; ShiftTimes "Time differences for switch [tA, tB, tC] (s) :"
      mask init: same as SPGF_FSK_0000_R2022b/Feed/Q/breaker
      mask Display:
      | % port_label('input',1,'Iabc');
      | 
      | port_label('lconn',1,'A');
      | port_label('lconn',2,'B');
      | port_label('lconn',3,'C');
      | 
      | port_label('rconn',1,'a');
      | port_label('rconn',2,'b');
      | port_label('rconn',3,'c');
      | 
      | disp('   Q    ');
  meas : Subsystem
  shunt : Subsystem
  A : PMIOPort  Side=Right
  B : PMIOPort  Port=2  Side=Right
  C : PMIOPort  Port=3  Side=Right
  a : PMIOPort  Port=4  Side=Left
  b : PMIOPort  Port=5  Side=Left
  c : PMIOPort  Port=6  Side=Left
  connections:
  shunt/LConn3 -- breaker/LConn3 -- C/RConn1
  shunt/LConn2 -- breaker/LConn2 -- B/RConn1
  A/RConn1 -- breaker/LConn1 -- shunt/LConn1
  meas/RConn1 -- a/RConn1
  meas/RConn2 -- b/RConn1
  meas/RConn3 -- c/RConn1
  meas/LConn3 -- breaker/RConn3 -- shunt/RConn3
  meas/LConn2 -- breaker/RConn2 -- shunt/RConn2
  meas/LConn1 -- breaker/RConn1 -- shunt/RConn1

== system SPGF_FSK_0000_R2022b/W21/concentrated ==
  Ccs/1 : spsSeriesRLCBranchLib/Series RLC Branch  LConnTagsString=__new0  RConnTagsString=__new0  BranchType=C  Resistance=190  Inductance=1e-3  SetiL0=off  InitialCurrent=0  Capacitance=-C_matrix(1,2)/2  Setx0=off  InitialVoltage=0  Measurements=None
  Ccs/2 : spsSeriesRLCBranchLib/Series RLC Branch  LConnTagsString=__new0  RConnTagsString=__new0  BranchType=C  Resistance=190  Inductance=1e-3  SetiL0=off  InitialCurrent=0  Capacitance=-C_matrix(1,2)/2  Setx0=off  InitialVoltage=0  Measurements=None
  Ccs2/1 : spsSeriesRLCBranchLib/Series RLC Branch  LConnTagsString=__new0  RConnTagsString=__new0  BranchType=C  Resistance=190  Inductance=1e-3  SetiL0=off  InitialCurrent=0  Capacitance=-C_matrix(3,4)/2  Setx0=off  InitialVoltage=0  Measurements=None
  Ccs2/2 : spsSeriesRLCBranchLib/Series RLC Branch  LConnTagsString=__new0  RConnTagsString=__new0  BranchType=C  Resistance=190  Inductance=1e-3  SetiL0=off  InitialCurrent=0  Capacitance=-C_matrix(3,4)/2  Setx0=off  InitialVoltage=0  Measurements=None
  Ccs2/3 : spsSeriesRLCBranchLib/Series RLC Branch  LConnTagsString=__new0  RConnTagsString=__new0  BranchType=R  Resistance=-Rg_matrix(3,4)*2  Inductance=1e-3  SetiL0=off  InitialCurrent=0  Capacitance=Rg_matrix(3,4)*2  Setx0=off  InitialVoltage=0  Measurements=None
  Ccs2/4 : spsSeriesRLCBranchLib/Series RLC Branch  LConnTagsString=__new0  RConnTagsString=__new0  BranchType=R  Resistance=-Rg_matrix(3,4)*2  Inductance=1e-3  SetiL0=off  InitialCurrent=0  Capacitance=Rg_matrix(3,4)*2  Setx0=off  InitialVoltage=0  Measurements=None
  Ccs3/1 : spsSeriesRLCBranchLib/Series RLC Branch  LConnTagsString=__new0  RConnTagsString=__new0  BranchType=C  Resistance=190  Inductance=1e-3  SetiL0=off  InitialCurrent=0  Capacitance=-C_matrix(5,6)/2  Setx0=off  InitialVoltage=0  Measurements=None
  Ccs3/2 : spsSeriesRLCBranchLib/Series RLC Branch  LConnTagsString=__new0  RConnTagsString=__new0  BranchType=C  Resistance=190  Inductance=1e-3  SetiL0=off  InitialCurrent=0  Capacitance=-C_matrix(5,6)/2  Setx0=off  InitialVoltage=0  Measurements=None
  Ccs3/3 : spsSeriesRLCBranchLib/Series RLC Branch  LConnTagsString=__new0  RConnTagsString=__new0  BranchType=R  Resistance=-Rg_matrix(5,6)*2  Inductance=1e-3  SetiL0=off  InitialCurrent=0  Capacitance=-C_matrix(5,6)/2  Setx0=off  InitialVoltage=0  Measurements=None
  Ccs3/4 : spsSeriesRLCBranchLib/Series RLC Branch  LConnTagsString=__new0  RConnTagsString=__new0  BranchType=R  Resistance=-Rg_matrix(5,6)*2  Inductance=1e-3  SetiL0=off  InitialCurrent=0  Capacitance=-C_matrix(5,6)/2  Setx0=off  InitialVoltage=0  Measurements=None
  Csg/2 : spsSeriesRLCBranchLib/Series RLC Branch  LConnTagsString=__new0  RConnTagsString=__new0  BranchType=C  Resistance=190  Inductance=1e-3  SetiL0=off  InitialCurrent=0  Capacitance=( C_matrix(1,2) + C_matrix(2,2) )/2  Setx0=off  InitialVoltage=0  Measurements=None
  Csg1/1 : spsSeriesRLCBranchLib/Series RLC Branch  LConnTagsString=__new0  RConnTagsString=__new0  BranchType=C  Resistance=190  Inductance=1e-3  SetiL0=off  InitialCurrent=0  Capacitance=( C_matrix(1,2) + C_matrix(2,2) )/2  Setx0=off  InitialVoltage=0  Measurements=None
  Csg2/1 : spsSeriesRLCBranchLib/Series RLC Branch  LConnTagsString=__new0  RConnTagsString=__new0  BranchType=C  Resistance=190  Inductance=1e-3  SetiL0=off  InitialCurrent=0  Capacitance=( C_matrix(3,4) + C_matrix(4,4) )/2  Setx0=off  InitialVoltage=0  Measurements=None
  Csg2/2 : spsSeriesRLCBranchLib/Series RLC Branch  LConnTagsString=__new0  RConnTagsString=__new0  BranchType=C  Resistance=190  Inductance=1e-3  SetiL0=off  InitialCurrent=0  Capacitance=( C_matrix(3,4) + C_matrix(4,4) )/2  Setx0=off  InitialVoltage=0  Measurements=None
  Csg3/1 : spsSeriesRLCBranchLib/Series RLC Branch  LConnTagsString=__new0  RConnTagsString=__new0  BranchType=C  Resistance=190  Inductance=1e-3  SetiL0=off  InitialCurrent=0  Capacitance=( C_matrix(5,6) + C_matrix(6,6) ) /2  Setx0=off  InitialVoltage=0  Measurements=None
  Csg3/2 : spsSeriesRLCBranchLib/Series RLC Branch  LConnTagsString=__new0  RConnTagsString=__new0  BranchType=C  Resistance=190  Inductance=1e-3  SetiL0=off  InitialCurrent=0  Capacitance=( C_matrix(5,6) + C_matrix(6,6) ) /2  Setx0=off  InitialVoltage=0  Measurements=None
  Ground{1..4} (4 alike) : spsGroundLib/Ground  LConnTagsString=a
  RL : spsMutualInductanceLib/Mutual Inductance  LConnTagsString=a|b|c|L4|L5|L6  RConnTagsString=A|B|C|R4|R5|R6  TypeOfMutual=Generalized mutual inductance  NumberOfWindings=6  SelfImpedance1=[1.1 1.1e-03]  SelfImpedance2=[ 1.1 1.1e-03]  ThreeWindings=on  SelfImpedance3=[ 1.1 1.1e-03]  MutualImpedance=[1.0 1.0e-03]  InductanceMatrix=L_matrix  ResistanceMatrix=R_matrix  Measurements=None
      settings: LibrarySourceBlock=sps_lib/Passives/Mutual Inductance
  Rcs*2 : spsSeriesRLCBranchLib/Series RLC Branch  LConnTagsString=__new0  RConnTagsString=__new0  BranchType=R  Resistance=-Rg_matrix(1,2)*2  Inductance=1e-3  SetiL0=off  InitialCurrent=0  Capacitance=Rg_matrix(1,2)*2  Setx0=off  InitialVoltage=0  Measurements=None
  Rgcs1/1 : spsSeriesRLCBranchLib/Series RLC Branch  LConnTagsString=__new0  RConnTagsString=__new0  BranchType=R  Resistance=-Rg_matrix(1,2)*2  Inductance=1e-3  SetiL0=off  InitialCurrent=0  Capacitance=Rg_matrix(1,2)*2  Setx0=off  InitialVoltage=0  Measurements=None
  Rgsg1/1 : spsSeriesRLCBranchLib/Series RLC Branch  LConnTagsString=__new0  RConnTagsString=__new0  BranchType=R  Resistance=(Rg_matrix(4,4)+Rg_matrix(3,4))*2  Inductance=1e-3  SetiL0=off  InitialCurrent=0  Capacitance=Rg_matrix(1,2)*2  Setx0=off  InitialVoltage=0  Measurements=None
  Rgsg1/2 : spsSeriesRLCBranchLib/Series RLC Branch  LConnTagsString=__new0  RConnTagsString=__new0  BranchType=R  Resistance=(Rg_matrix(2,2)+Rg_matrix(1,2))*2  Inductance=1e-3  SetiL0=off  InitialCurrent=0  Capacitance=Rg_matrix(1,2)*2  Setx0=off  InitialVoltage=0  Measurements=None
  Rgsg1/3 : spsSeriesRLCBranchLib/Series RLC Branch  LConnTagsString=__new0  RConnTagsString=__new0  BranchType=R  Resistance=(Rg_matrix(4,4)+Rg_matrix(3,4))*2  Inductance=1e-3  SetiL0=off  InitialCurrent=0  Capacitance=Rg_matrix(1,2)*2  Setx0=off  InitialVoltage=0  Measurements=None
  Rgsg1/4 : spsSeriesRLCBranchLib/Series RLC Branch  LConnTagsString=__new0  RConnTagsString=__new0  BranchType=R  Resistance=(Rg_matrix(2,2)+Rg_matrix(1,2))*2  Inductance=1e-3  SetiL0=off  InitialCurrent=0  Capacitance=Rg_matrix(1,2)*2  Setx0=off  InitialVoltage=0  Measurements=None
  Rsg*2 : spsSeriesRLCBranchLib/Series RLC Branch  LConnTagsString=__new0  RConnTagsString=__new0  BranchType=R  Resistance=(Rg_matrix(6,6)+Rg_matrix(5,6))*2  Inductance=1e-3  SetiL0=off  InitialCurrent=0  Capacitance=Rg_matrix(1,2)*2  Setx0=off  InitialVoltage=0  Measurements=None
  Rsg1/1 : spsSeriesRLCBranchLib/Series RLC Branch  LConnTagsString=__new0  RConnTagsString=__new0  BranchType=R  Resistance=(Rg_matrix(6,6)+Rg_matrix(5,6))*2  Inductance=1e-3  SetiL0=off  InitialCurrent=0  Capacitance=Rg_matrix(1,2)*2  Setx0=off  InitialVoltage=0  Measurements=None
  A : PMIOPort  Side=Left
  B : PMIOPort  Port=2  Side=Left
  C : PMIOPort  Port=3  Side=Left
  a : PMIOPort  Port=4  Side=Right
  b : PMIOPort  Port=5  Side=Right
  c : PMIOPort  Port=6  Side=Right
  connections:
  RL/LConn6 -- Ground3/LConn1 -- Rgsg1/2/LConn1 -- Csg/2/LConn1 -- Rcs*2/LConn1 -- Ccs/2/LConn1 -- RL/LConn2 -- RL/LConn4 -- Rgsg1/1/LConn1 -- Csg2/2/LConn1 -- Ccs2/3/LConn1 -- Ccs2/2/LConn1 -- Rsg*2/LConn1 -- Csg3/2/LConn1 -- Ccs3/3/LConn1 -- Ccs3/2/LConn1
  Rsg1/1/RConn1 -- Rgsg1/3/RConn1 -- Rgsg1/4/RConn1 -- Csg3/1/RConn1 -- Csg2/1/RConn1 -- Ground2/LConn1 -- Csg1/1/RConn1
  Rgsg1/3/LConn1 -- Ccs2/4/LConn1 -- Csg2/1/LConn1 -- Ccs2/1/LConn1 -- RL/RConn4 -- Rgsg1/4/LConn1 -- Rgcs1/1/LConn1 -- Csg1/1/LConn1 -- Ccs/1/LConn1 -- RL/RConn2 -- Ground4/LConn1 -- RL/RConn6 -- Ccs3/1/LConn1 -- Rsg1/1/LConn1 -- Ccs3/4/LConn1 -- Csg3/1/LConn1
  Rsg*2/RConn1 -- Rgsg1/1/RConn1 -- Rgsg1/2/RConn1 -- Csg3/2/RConn1 -- Csg2/2/RConn1 -- Ground1/LConn1 -- Csg/2/RConn1
  a/RConn1 -- RL/RConn1 -- Rgcs1/1/RConn1 -- Ccs/1/RConn1
  b/RConn1 -- RL/RConn3 -- Ccs2/4/RConn1 -- Ccs2/1/RConn1
  Ccs3/1/RConn1 -- c/RConn1 -- RL/RConn5 -- Ccs3/4/RConn1
  RL/LConn1 -- A/RConn1 -- Rcs*2/RConn1 -- Ccs/2/RConn1
  RL/LConn3 -- B/RConn1 -- Ccs2/3/RConn1 -- Ccs2/2/RConn1
  Ccs3/2/RConn1 -- C/RConn1 -- RL/LConn5 -- Ccs3/3/RConn1
